simulink model "class18_simu"  (R2025b)
settings: Solver=VariableStepAuto  StartTime=0.0  StopTime=100  RelTol=1e-3
values from neighbouring files (symbols this model uses):
  A = [1 0;     0 1]    [Obs_temp.m]    (also in class10.m = [0       1              0                  0; class11.m = [0 1 0 0; class12.m = [0 1; -k/m -c/m]; class13.m = [0 1; -k/m -c/m])
  B = 1    [Obs_temp.m]    (also in class10.m = [0; class11.m = [0; 1/M; 0; s*1/(M*L)]; class12.m = [0; 1/m]; class13.m = [0; 1/m])
  C = [1 0]    [Obs_temp.m]    (also in class12.m; class13.m; class14.m; class15.m)
  K = lqr(A,B,Q,R)    [class10.m]    (also in class11.m; class21.m; class5.m = [0 0 1]*inv(cm)*phi_A; class8.m = place(A,B,p))
  x0 = [-1,0]    [Obs_temp.m]    (also in class10.m = [-4; 0; pi+deg2rad(10); 0]; class11.m = [0;0;pi+1; 0]; class14.m = [-2,0,-10,-1]; class15.m = [-2; 0; 100; 100;])
undefined symbols (not defined in the file or in its folder): x0_o
settings Model: Creator=anish  LastModifiedBy=anish

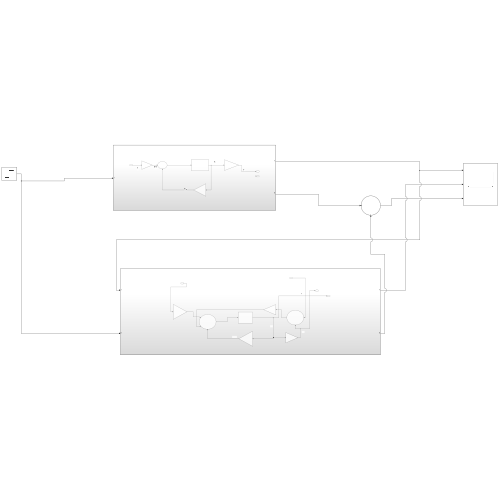
[thumbnail: Simulink's stored preview of the top-level diagram]
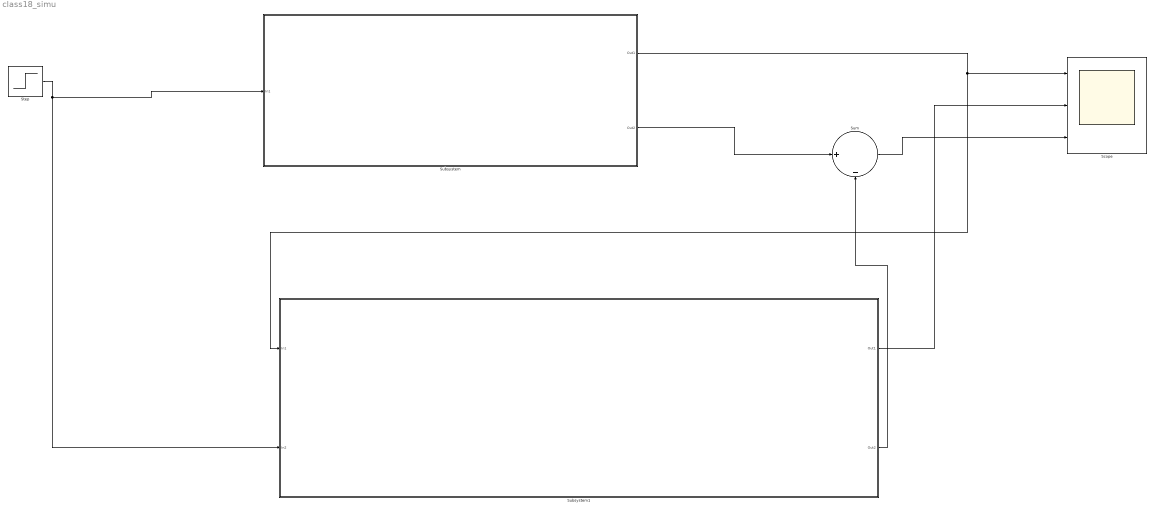
== system class18_simu ==
  Scope : Scope  NumInputPorts=3
      settings: SampleTime=0.01  ActiveDisplayYMinimum=-0.51546839933148669  ActiveDisplayYMaximum=0.61373667113329322
  Step : Step  SampleTime=0
  Subsystem : Subsystem
  Subsystem1 : Subsystem
  Sum : Sum  Inputs=|+-
  wires:
  Subsystem1/1(Out1) -> Scope/2
  Subsystem/1(Out1) -> Subsystem1/1(In1), Scope/1
  Step/1 -> Subsystem/1(In1), Subsystem1/2(In2)
  Subsystem/2(Out2) -> Sum/1
  Subsystem1/2(Out2) -> Sum/2
  Sum/1 -> Scope/3

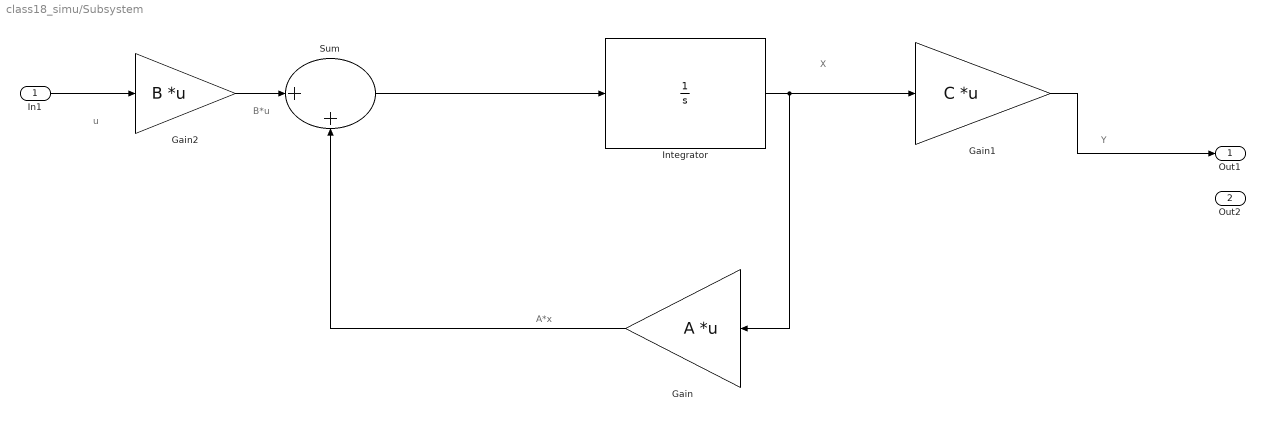
== system class18_simu/Subsystem ==
  note: Y
  note: X
  note: A*x
  note: u
  note: B*u
  In1 : Inport
  Gain : Gain  Gain=A  Multiplication=Matrix(K*u)
  Gain1 : Gain  Gain=C  Multiplication=Matrix(K*u)
  Gain2 : Gain  Gain=B  Multiplication=Matrix(K*u)
  Integrator : Integrator  InitialCondition=x0
  Sum : Sum  Inputs=|++
  Out1 : Outport
  Out2 : Outport  Port=2
  wires:
  In1/1 -> Gain2/1
  Gain/1 -> Sum/2
  Gain1/1 -> Out1/1
  Sum/1 -> Integrator/1
  Gain2/1 -> Sum/1
  Integrator/1 -> Gain1/1, Gain/1

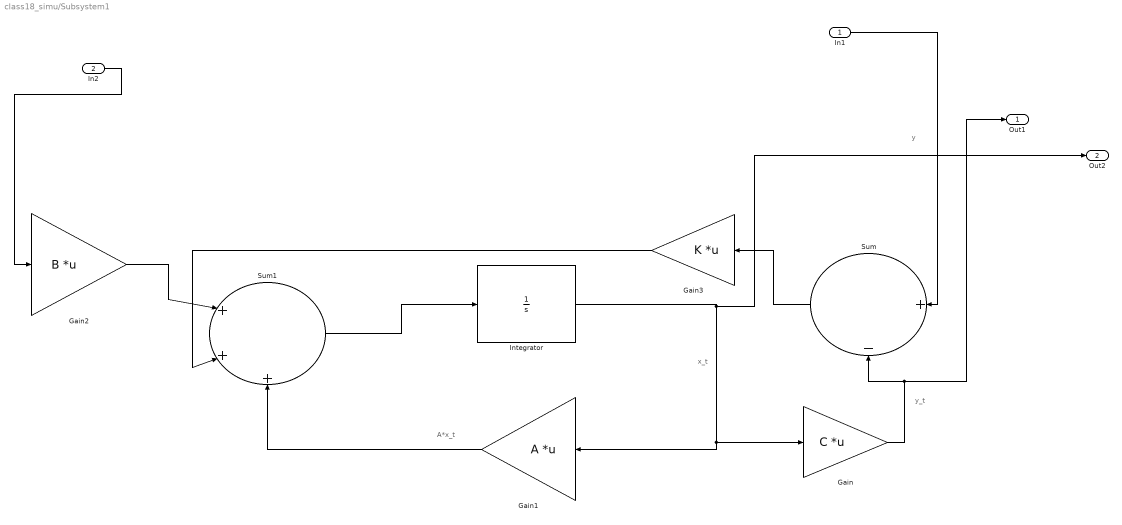
== system class18_simu/Subsystem1 ==
  note: y
  note: y_t
  note: x_t
  note: A*x_t
  In1 : Inport
  In2 : Inport  Port=2
  Gain : Gain  Gain=C  Multiplication=Matrix(K*u) (u vector)
  Gain1 : Gain  Gain=A  Multiplication=Matrix(K*u) (u vector)
  Gain2 : Gain  Gain=B  Multiplication=Matrix(K*u) (u vector)
  Gain3 : Gain  Gain=K  Multiplication=Matrix(K*u) (u vector)
  Integrator : Integrator  InitialCondition=x0_o
  Sum : Sum  Inputs=|+-
  Sum1 : Sum  Inputs=|+++
  Out1 : Outport
  Out2 : Outport  Port=2
  wires:
  Gain2/1 -> Sum1/1
  In2/1 -> Gain2/1
  In1/1 -> Sum/1
  Gain1/1 -> Sum1/3
  Gain3/1 -> Sum1/2
  Sum1/1 -> Integrator/1
  Sum/1 -> Gain3/1
  Gain/1 -> Out1/1, Sum/2
  Integrator/1 -> Out2/1, Gain/1, Gain1/1
